simulink model "sgMdl_IO425_LVDTResolverEmulation"  (R2024b)
settings: Solver=FixedStepAuto  StartTime=0.0  StopTime=inf  RelTol=1e-3  EnableMultiTasking=on
libraries: speedgoatlib_IO425 x2, simulink x1
Description:
  | IO425 - LVDT/RVDT/Resolver Emulation
settings Model: ModifiedByFormat=Speedgoat  Creator=Speedgoat  LastModifiedBy=Speedgoat
settings SolverCC: ConcurrentTasks=on  AlgebraicLoopSolver=TrustRegion  PositivePriorityOrder=on  InsertRTBMode=Never (minimum delay)
settings DataIOCC: LimitDataPoints=on  SaveFormat=Array  SignalLoggingSaveFormat=ModelDataLogs  ReturnWorkspaceOutputs=off
settings OptimizationCC: BlockReduction=off  OptimizeBlockIOStorage=off  BufferReuse=off  GlobalBufferReuse=off  ExpressionFolding=off  ExpressionDepthLimit=2147483647  LocalBlockOutputs=off  OptimizeDataStoreBuffers=off  BusAssignmentInplaceUpdate=off
settings DebuggingCC: UnderspecifiedInitializationDetection=Classic  MergeDetectMultiDrivingBlocksExec=none  SolverPrmCheckMsg=warning  TasksWithSamePriorityMsg=none  FcnCallInpInsideContextMsg=warning  StateNameClashWarn=warning  SFUnexpectedBacktrackingDiag=warning  SFNoUnconditionalDefaultTransitionDiag=warning  SFExecutionAtInitializationDiag=none  ArithmeticOperatorsInVariantConditions=warning
settings HardwareCC: ProdBitPerLong=64  ProdLongLongMode=on  ProdHWDeviceType=Intel->x86-64 (Linux 64)
settings ModelReferenceCC: EnableRefExpFcnMdlSchedulingChecks=on  PropagateSignalLabelsOutOfModel=off
settings SFSimCC: SimUseLocalCustomCode=off  CustomCodeUndefinedFunction=UseInterfaceOnly
settings RTWCC: Description=Speedgoat Real-Time Target Machine  SystemTargetFile=speedgoat.tlc  TemplateMakefile=slrealtime_default_tmf  RTWUseLocalCustomCode=off  Toolchain=Simulink Real-Time Toolchain  BuildConfiguration=Faster Runs  TargetLang=C++  GPUComputeCapability=3.5  DLArmComputeVersion=19.05
settings CodeAppCC: StateflowObjectComments=on
settings SimulinkRealTimeTargetCC: SubcomponentCodeInterfacePackaging=Reusable function  InstructionSetFMA=off  LogToMDFFile=off  SLRTFileLogMaxRuns=10  UseGCCFastMath=on
settings ConfigComp: CovMetricSettings=dw  CovSaveCumulativeToWorkspaceVar=on  CovSaveSingleToWorkspaceVar=on  CovExternalEMLEnable=off  CovSFcnEnable=off  CovBoundaryAbsTol=1.0e-5

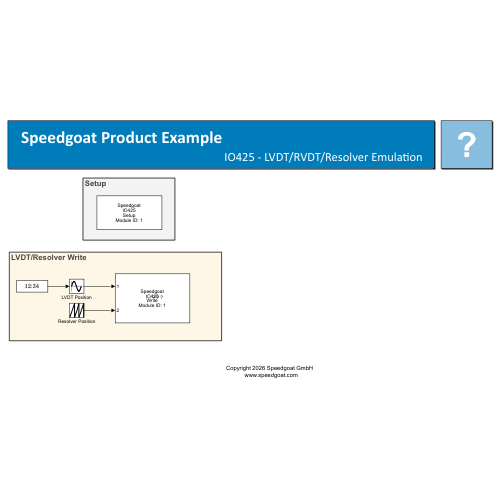
[thumbnail: Simulink's stored preview of the top-level diagram]
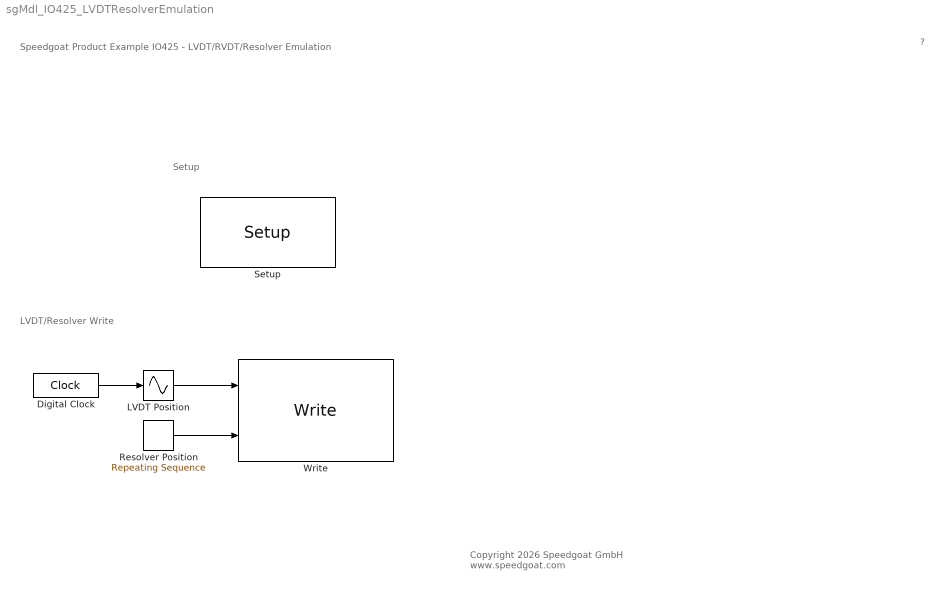
== system sgMdl_IO425_LVDTResolverEmulation ==
  note: Setup
  note: LVDT/Resolver Write
  note: Speedgoat Product Example
      | IO425 - LVDT/RVDT/Resolver Emulation
  note: ?
  note: Copyright 2026 Speedgoat GmbH
      |  www.speedgoat.com
  Digital Clock : DigitalClock
  LVDT Position : Sin  TimeSource=Use external signal  Amplitude=100  Frequency=pi/2  SampleTime=0.1
  Resolver Position : simulink/Sources/Repeating Sequence  rep_seq_t=[0 2.5 5]  rep_seq_y=[0 180 360]
  "Setup " : speedgoatlib_IO425/Setup   parModuleId=1  parPciSlot=-1  parCh1=4-Wire LVDT/RVDT  parCh2=Disabled  parCh3=Resolver  parCh4=Disabled  parOutVoltage=[3 5]  parPhaseA=[0 0]  parPhaseB=[0 0]  parInvertA=[0 0]  parInvertB=[0 0]  parExcMode=[1 1]  parExcFreq=[2e3 10e3]  parSampleBuffer=[]  parEnExcCal=off  parExcGain=[100 100]  parPosLVDT=[0]  parResetLVDT=[0]  parNullOffset=[50]  parPosResolver=[45]  parResetResolver=[1]
      settings: SourceProductName=Simulink Real-Time: Speedgoat I/O Blockset
  "Write " : speedgoatlib_IO425/Write   parModuleId=1  parTs=-1  parPciSlot=-1  parChannels=[1 3]  parMode=[1 3]  parShowStatus=off  parShowInVoltage=off  parShowInFreq=off  parShowPos=off  parEnInCtrl=off  parEnOutACtrl=off  parEnOutBCtrl=off
      settings: SourceProductName=Simulink Real-Time: Speedgoat I/O Blockset
  wires:
  Resolver Position/1 -> "Write "/2
  LVDT Position/1 -> "Write "/1
  Digital Clock/1 -> LVDT Position/1
